simulink model "P3_BiHPF "  (R2020b)
settings: Solver=VariableStepAuto  StartTime=0.0  StopTime=10.0  RelTol=1e-3
model workspace (MAT data in the model file):
  a0 = 1
  a1 = 0.1584
  b0 = 0.5792
  b1 = -0.5792
  h2r = 6.28318530718
settings Model: OrderedModelArguments=off  Creator=mluser  LastModifiedBy=mluser

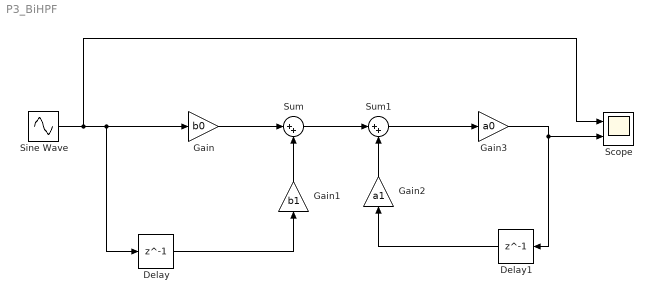
== system P3_BiHPF  ==
  Delay : Delay  DelayLength=1
  Delay1 : Delay  DelayLength=1
  Gain : Gain  Gain=b0
  Gain1 : Gain  Gain=b1
  Gain2 : Gain  Gain=a1
  Gain3 : Gain  Gain=a0
  Scope : Scope  NumInputPorts=2
  Sine Wave : Sin  Frequency=700*h2r  SampleTime=0
  Sum : Sum  Inputs=|++
  Sum1 : Sum  Inputs=|++
  wires:
  Gain/1 -> Sum/1
  Gain1/1 -> Sum/2
  Delay/1 -> Gain1/1
  Sum/1 -> Sum1/1
  Gain2/1 -> Sum1/2
  Sum1/1 -> Gain3/1
  Delay1/1 -> Gain2/1
  Gain3/1 -> Delay1/1, Scope/2
  Sine Wave/1 -> Scope/1, Delay/1, Gain/1
